simulink library "arducopter_library"  (R2016a)
settings: Solver=ode45  StartTime=0.0  StopTime=10.0  RelTol=1e-3
undefined symbols (not defined in the file): P, use_ff
libraries: simulink x1, arducopter_library x1
settings Model: Creator=anne  LastModifiedBy=anne
settings DataIOCC: LimitDataPoints=on
settings DebuggingCC: AllowSymbolicDim=off

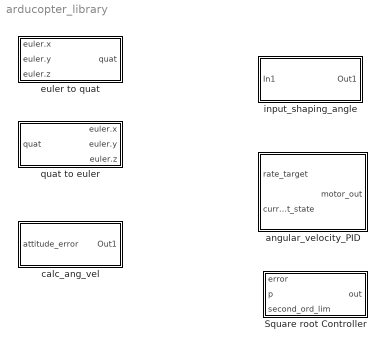
== system arducopter_library ==
  Square root Controller : Subsystem
  angular_velocity_PID : Subsystem  mask(The pid controller for angular velocity){P_rate=0, I_rate=0, D_rate=0, N=0}
      mask prompts: P_rate "P rate"; I_rate "I rate"; D_rate "D rate"; N "Filter Hz"
      mask DialogControl Control3 Prompt: Angular Velocity PID
  calc_ang_vel : Subsystem
  euler to quat : Subsystem
  input_shaping_angle : Subsystem
  quat to euler : Subsystem

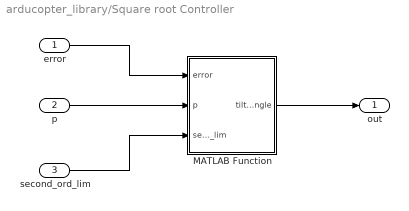
== system arducopter_library/Square root Controller ==
  error : Inport
  p : Inport  Port=2
  second_ord_lim : Inport  Port=3
  MATLAB Function : MATLAB Function  TreatAsAtomicUnit=on
  out : Outport
  wires:
  error/1 -> MATLAB Function/1(error)
  p/1 -> MATLAB Function/2(p)
  second_ord_lim/1 -> MATLAB Function/3(second_ord_lim)
  MATLAB Function/1(tilt_angle) -> out/1

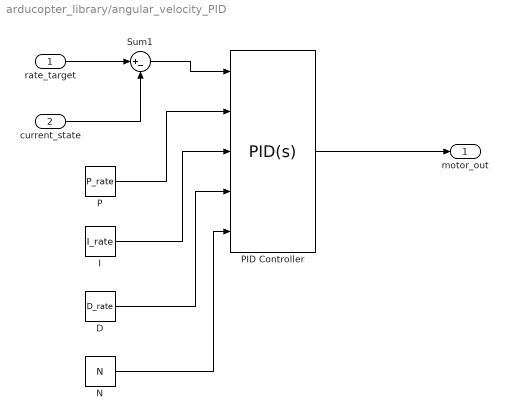
== system arducopter_library/angular_velocity_PID ==
  rate_target : Inport
  current_state : Inport  Port=2
  D : Constant  Value=D_rate
  I : Constant  Value=I_rate
  N : Constant  Value=N
  P : Constant  Value=P_rate
  PID Controller : simulink/Continuous/PID Controller  Controller=PID  TimeDomain=Continuous-time  SampleTime=-1  IntegratorMethod=Forward Euler  FilterMethod=Forward Euler  Form=Parallel  UseFilter=on  ControllerParametersSource=external  P=1  I=1  D=0  N=100  InitialConditionSource=internal  InitialConditionForIntegrator=0  InitialConditionForFilter=0  ExternalReset=none  LimitOutput=off  UpperSaturationLimit=inf  LowerSaturationLimit=-inf  LinearizeAsGain=on  AntiWindupMode=none  Kb=1  TrackingMode=off  Kt=1  PParamMin=[]  PParamMax=[]  IParamMin=[]  IParamMax=[]  DParamMin=[]  DParamMax=[]  NParamMin=[]  NParamMax=[]  KbParamMin=[]  KbParamMax=[]  KtParamMin=[]  KtParamMax=[]  POutMin=[]  POutMax=[]  IOutMin=[]  IOutMax=[]  DOutMin=[]  DOutMax=[]  NOutMin=[]  NOutMax=[]  KbOutMin=[]  KbOutMax=[]  KtOutMin=[]  KtOutMax=[]  IntegratorOutMin=[]  IntegratorOutMax=[]  FilterOutMin=[]  FilterOutMax=[]  SumOutMin=[]  SumOutMax=[]  SumI1OutMin=[]  SumI1OutMax=[]  SumI2OutMin=[]  SumI2OutMax=[]  SumI3OutMin=[]  SumI3OutMax=[]  SumDOutMin=[]  SumDOutMax=[]  SaturationOutMin=[]  SaturationOutMax=[]  IntegratorContinuousStateAttributes=''  IntegratorStateMustResolveToSignalObject=off  IntegratorRTWStateStorageClass=Auto  FilterContinuousStateAttributes=''  FilterStateMustResolveToSignalObject=off  FilterRTWStateStorageClass=Auto  DifferentiatorICPrevScaledInput=0  DifferentiatorOutMin=[]  DifferentiatorOutMax=[]
  Sum1 : Sum  Inputs=|+-
  motor_out : Outport
  wires:
  rate_target/1 -> Sum1/1
  Sum1/1 -> PID Controller/1
  current_state/1 -> Sum1/2
  P/1 -> PID Controller/2
  I/1 -> PID Controller/3
  D/1 -> PID Controller/4
  N/1 -> PID Controller/5
  PID Controller/1 -> motor_out/1

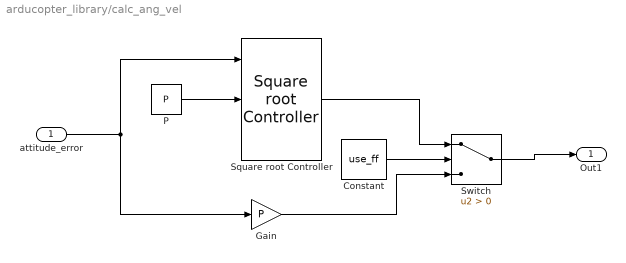
== system arducopter_library/calc_ang_vel ==
  attitude_error : Inport
  Constant : Constant  Value=use_ff
  Gain : Gain  Gain=P
  P : Constant  Value=P
  Square root Controller : arducopter_library/Square root Controller  SystemSampleTime=-1
  Switch : Switch  Criteria=u2 > Threshold
  Out1 : Outport
  wires:
  Square root Controller/1 -> Switch/1
  attitude_error/1 -> Square root Controller/1, Gain/1
  Gain/1 -> Switch/3
  Switch/1 -> Out1/1
  Constant/1 -> Switch/2
  P/1 -> Square root Controller/2

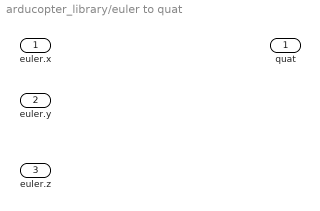
== system arducopter_library/euler to quat ==
  euler.x : Inport
  euler.y : Inport  Port=2
  euler.z : Inport  Port=3
  quat : Outport

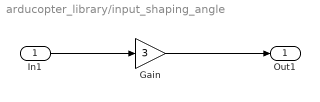
== system arducopter_library/input_shaping_angle ==
  In1 : Inport
  Gain : Gain  Gain=3
  Out1 : Outport
  wires:
  In1/1 -> Gain/1
  Gain/1 -> Out1/1

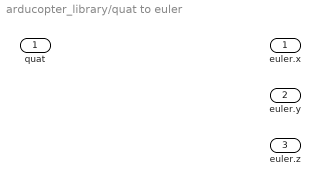
== system arducopter_library/quat to euler ==
  quat : Inport
  euler.x : Outport
  euler.y : Outport  Port=2
  euler.z : Outport  Port=3

== matlab function arducopter_library/Square root Controller/MATLAB Function ==
  data: error input; tilt_angle output; p input; second_ord_lim input
function tilt_angle = sqr_ctrl(error, p, second_ord_lim)
    if second_ord_lim <= 0 || p==0
        tilt_angle = error * p;
        return
    end
    
    linear_dist = second_ord_lim/(p^2);
    
    if error > linear_dist
        tilt_angle = sqrt(2*second_ord_lim*(error-(linear_dist/2)));
        return
    elseif error < -linear_dist
        tilt_angle = sqrt(2*second_ord_lim*(-error-(linear_dist/2)));
        return
    else
        tilt_angle = error * p;
        return
    end
end
